simulink model "MixingTank_KalmanFilter_Simulink2017b"  (R2018b)
settings: Solver=ode4  StartTime=0.0  StopTime=SIM_TIME  FixedStep=STEP_SIZE  RelTol=1e-3
undefined symbols (not defined in the file): At, Av, C_kf, Cv, F_kf, G_kf, kh, kt, kv, L_kf, Ts, u0, V2d, x0, x0hat, y0
settings Model: Creator=Roberto  LastModifiedBy=Roberto
settings SFSimCC: SimUseLocalCustomCode=off
settings RTWCC: RTWUseLocalCustomCode=off

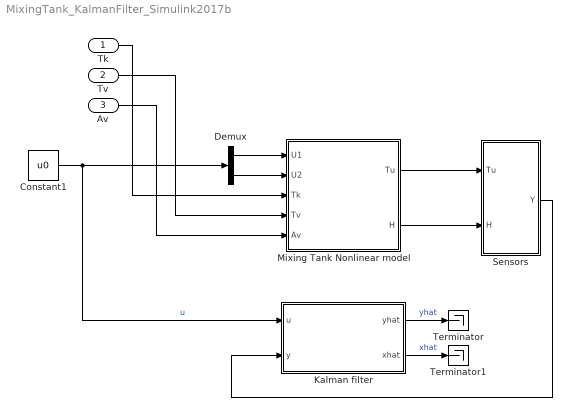
== system MixingTank_KalmanFilter_Simulink2017b ==
  Tk : Inport
  Tv : Inport  Port=2
  Av : Inport  Port=3
  Constant1 : Constant  Value=u0
  Demux : Demux  Outputs=2
  Kalman filter : Subsystem
  Mixing Tank Nonlinear model : Subsystem
  Sensors : Subsystem
  Terminator : Terminator
  Terminator1 : Terminator
  wires:
  Tk/1 -> Mixing Tank Nonlinear model/3(Tk)
  Tv/1 -> Mixing Tank Nonlinear model/4(Tv)
  Av/1 -> Mixing Tank Nonlinear model/5(Av)
  Demux/2 -> Mixing Tank Nonlinear model/2(U2)
  Demux/1 -> Mixing Tank Nonlinear model/1(U1)
  Constant1/1 -> Kalman filter/1(u), Demux/1  "u"
  Kalman filter/2(xhat) -> Terminator1/1  "xhat"
  Kalman filter/1(yhat) -> Terminator/1  "yhat"
  Mixing Tank Nonlinear model/1(Tu) -> Sensors/1(Tu)
  Mixing Tank Nonlinear model/2(H) -> Sensors/2(H)
  Sensors/1(Y) -> Kalman filter/2(y)

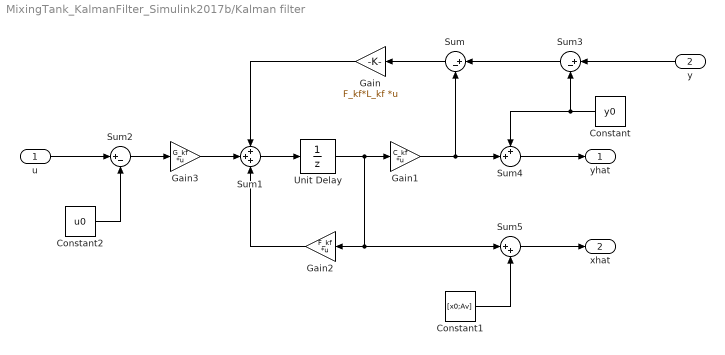
== system MixingTank_KalmanFilter_Simulink2017b/Kalman filter ==
  u : Inport
  y : Inport  Port=2
  Constant : Constant  Value=y0
  Constant1 : Constant  Value=[x0;Av]
  Constant2 : Constant  Value=u0
  Gain : Gain  Gain=F_kf*L_kf  Multiplication=Matrix(K*u) (u vector)
  Gain1 : Gain  Gain=C_kf  Multiplication=Matrix(K*u) (u vector)
  Gain2 : Gain  Gain=F_kf  Multiplication=Matrix(K*u) (u vector)
  Gain3 : Gain  Gain=G_kf  Multiplication=Matrix(K*u) (u vector)
  Sum : Sum  Inputs=|+-
  Sum1 : Sum  Inputs=+++
  Sum2 : Sum  Inputs=|+-
  Sum3 : Sum  Inputs=|+-
  Sum4 : Sum  Inputs=++|
  Sum5 : Sum  Inputs=|++
  Unit Delay : UnitDelay  InitialCondition=x0hat  SampleTime=-1
  yhat : Outport
  xhat : Outport  Port=2
  wires:
  Constant/1 -> Sum4/1, Sum3/2
  Gain3/1 -> Sum1/2
  Constant2/1 -> Sum2/2
  Sum3/1 -> Sum/1
  Gain/1 -> Sum1/1
  Sum/1 -> Gain/1
  Gain1/1 -> Sum4/2, Sum/2
  Unit Delay/1 -> Sum5/1, Gain2/1, Gain1/1
  Sum2/1 -> Gain3/1
  Gain2/1 -> Sum1/3
  Sum1/1 -> Unit Delay/1
  y/1 -> Sum3/1
  u/1 -> Sum2/1
  Constant1/1 -> Sum5/2
  Sum4/1 -> yhat/1
  Sum5/1 -> xhat/1

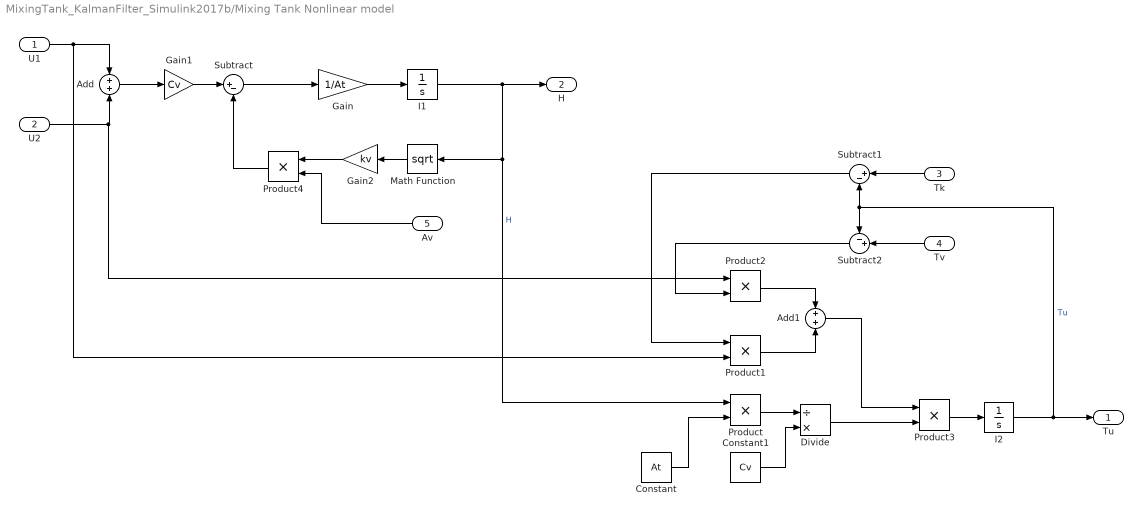
== system MixingTank_KalmanFilter_Simulink2017b/Mixing Tank Nonlinear model ==
  U1 : Inport
  U2 : Inport  Port=2
  Tk : Inport  Port=3
  Tv : Inport  Port=4
  Av : Inport  Port=5
  Add : Sum
  Add1 : Sum
  Constant : Constant  Value=At
  Constant1 : Constant  Value=Cv
  Divide : Product  Inputs=/*
  Gain : Gain  Gain=1/At
  Gain1 : Gain  Gain=Cv
  Gain2 : Gain  Gain=kv
  I1 : Integrator  Priority=1  InitialCondition=x0(1)  LimitOutput=on  LowerSaturationLimit=0
  I2 : Integrator  Priority=2  InitialCondition=x0(2)
  Math Function : Math  Operator=sqrt  SaturateOnIntegerOverflow=on
  Product{,1..4} (5 alike) : Product  RndMeth=Zero
  Subtract : Sum  Inputs=|+-
  Subtract1 : Sum  Inputs=|+-
  Subtract2 : Sum  Inputs=-+|
  Tu : Outport
  H : Outport  Port=2
  wires:
  Math Function/1 -> Gain2/1
  Gain2/1 -> Product4/1
  Product/1 -> Divide/1
  Subtract1/1 -> Product1/1
  Product3/1 -> I2/1
  I1/1 -> H/1, Math Function/1, Product/1  "H"
  Product4/1 -> Subtract/2
  Av/1 -> Product4/2
  Gain1/1 -> Subtract/1
  Add1/1 -> Product3/1
  Constant/1 -> Product/2
  Subtract2/1 -> Product2/2
  Tk/1 -> Subtract1/1
  Add/1 -> Gain1/1
  U1/1 -> Product1/2, Add/1
  Constant1/1 -> Divide/2
  Gain/1 -> I1/1
  U2/1 -> Product2/1, Add/2
  Subtract/1 -> Gain/1
  I2/1 -> Tu/1, Subtract2/1, Subtract1/2  "Tu"
  Tv/1 -> Subtract2/2
  Divide/1 -> Product3/2
  Product2/1 -> Add1/1
  Product1/1 -> Add1/2

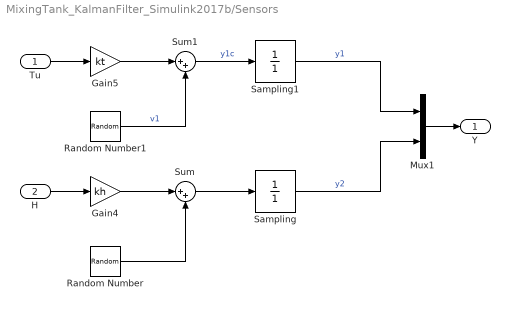
== system MixingTank_KalmanFilter_Simulink2017b/Sensors ==
  Tu : Inport
  H : Inport  Port=2
  Gain4 : Gain  Gain=kh
  Gain5 : Gain  Gain=kt
  Mux1 : Mux  Inputs=2
  Random Number : RandomNumber  Variance=V2d(2,2)  Seed=[951706]  SampleTime=Ts
  Random Number1 : RandomNumber  Variance=V2d(1,1)  Seed=[35498]  SampleTime=Ts
  Sampling : DiscreteTransferFcn  Denominator=[1]  SampleTime=Ts
  Sampling1 : DiscreteTransferFcn  Denominator=[1]  SampleTime=Ts
  Sum : Sum  Inputs=|++
  Sum1 : Sum  Inputs=|++
  Y : Outport
  wires:
  Random Number/1 -> Sum/2
  Gain5/1 -> Sum1/1
  Tu/1 -> Gain5/1
  Random Number1/1 -> Sum1/2  "v1"
  Gain4/1 -> Sum/1
  H/1 -> Gain4/1
  Mux1/1 -> Y/1
  Sum1/1 -> Sampling1/1  "y1c"
  Sampling1/1 -> Mux1/1  "y1"
  Sum/1 -> Sampling/1
  Sampling/1 -> Mux1/2  "y2"
